simulink subsystem "PvtSubSys_VSM_ISL"  (R2020b)
settings: Solver=VariableStepAuto  StartTime=0.0  StopTime=10.0  RelTol=1e-3
values from neighbouring files (symbols this model uses):
  P_VSM_ISL_AutoSpPpercentage = 0.1    [ISL.sldd]
  P_VSM_ISL_SLW_Warning_Time = 10.0    [ISL.sldd]
  P_VSM_ISL_SpdDOWNmaxDiff = 50.0    [ISL.sldd]
  P_VSM_ISL_SpdUPmaxDiff = 25.0    [ISL.sldd]
  P_VSM_ISL_SpdUPminDiff = 10.0    [ISL.sldd]
  P_VSM_ISL_TimeInformDis = 6.0    [ISL.sldd]
  P_VSM_ISL_TimeTakeOver = 30.0    [ISL.sldd]
undefined symbols (not defined in the file or in its folder): ACC_STATE, HWA_STATE, TJA_STATE
libraries: simulink x17
settings Model: Creator=GW00133806  LastModifiedBy=Cheng

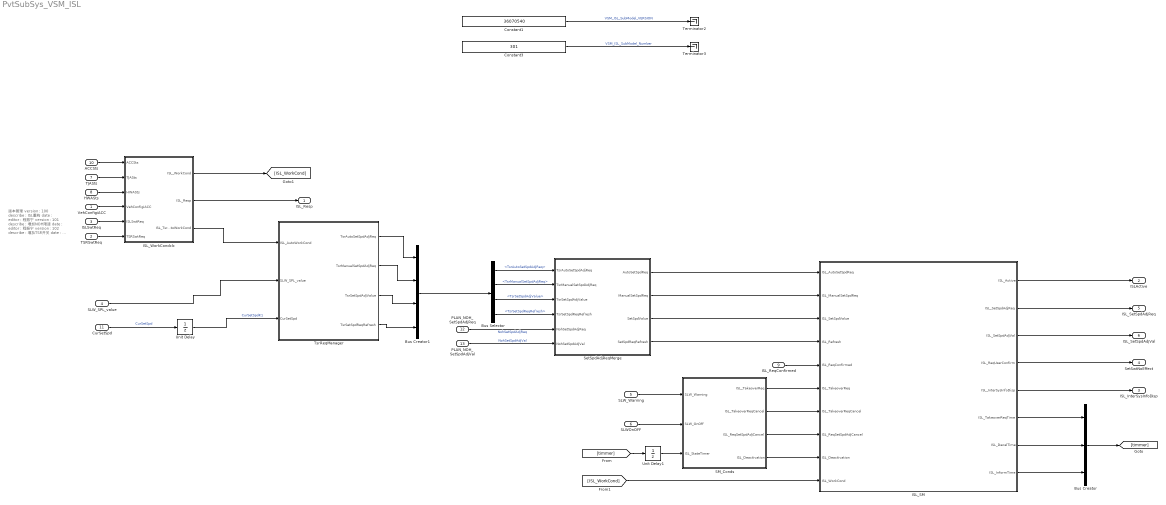
== system PvtSubSys_VSM_ISL ==
  note: 版本管理
      | version：100
      | describe：ISL重构
      | date：
      | editor：程振宁
      |
      | version：101
      | describe：增加NOH限速
      | date：
      | editor：程振宁
      |
      | version：102
      | describe：增加TSR开关
      | date：
      | editor：胡振国
  VehConfigiACC : Inport  OutDataTypeStr=uint8
  TSRSwtReq : Inport  Port=2
  ISLSwtReq : Inport  Port=3  OutDataTypeStr=boolean
  SLW_SPL_value : Inport  Port=4  OutDataTypeStr=uint8
  SLW_Warning : Inport  Port=5  OutDataTypeStr=boolean
  SLWOnOFF : Inport  Port=6  OutDataTypeStr=boolean
  TJASts : Inport  Port=7  OutDataTypeStr=Enum: TJA_STATE
  HWASts : Inport  Port=8  OutDataTypeStr=Enum: HWA_STATE
  ISL_ReqConfirmed : Inport  Port=9  OutDataTypeStr=boolean
  ACCSts : Inport  Port=10  OutDataTypeStr=Enum: ACC_STATE
  CurSetSpd : Inport  Port=11  OutDataTypeStr=single
  PLAN_NOH_SetSpdAdjReq : Inport  Port=12  OutDataTypeStr=boolean
  PLAN_NOH_SetSpdAdjVal : Inport  Port=13  OutDataTypeStr=uint8
  Bus Creator : BusCreator  Inputs=3
  Bus Creator1 : BusCreator  Inputs=4
  Bus Selector : BusSelector  OutputSignals=TsrAutoSetSpdAdjReq,TsrManualSetSpdAdjReq,TsrSetSpdAdjValue,TsrSetSpdReqRefresh
  Constant1 : Constant  Value=36070540  OutDataTypeStr=uint32
  Constant3 : Constant  Value=301  OutDataTypeStr=uint16
  ISL_SM : Stateflow chart  TreatAsAtomicUnit=on
  ISL_WorkCondclc : Subsystem
  SM_Conds : Subsystem
  SetSpdAdjReqMerge : Subsystem
  Terminator2 : Terminator
  Terminator3 : Terminator
  TsrReqManager : Subsystem
  Unit Delay : UnitDelay  SampleTime=-1  HasFrameUpgradeWarning=on
  Unit Delay1 : UnitDelay  SampleTime=-1  HasFrameUpgradeWarning=on
  ISL_Resp : Outport  OutDataTypeStr=boolean
  ISLActive : Outport  Port=2  OutDataTypeStr=boolean
  ISL_InterSysInfoDisp : Outport  Port=3  OutDataTypeStr=uint8
  SetSwtNoEffect : Outport  Port=4  OutDataTypeStr=boolean
  ISL_SetSpdAdjReq : Outport  Port=5  OutDataTypeStr=boolean
  ISL_SetSpdAdjVal : Outport  Port=6  OutDataTypeStr=uint8
  wires:
  Constant3/1 -> Terminator3/1  "VSM_ISL_SubModel_Number"
  Constant1/1 -> Terminator2/1  "VSM_ISL_SubModel_VERSION"
  TSRSwtReq/1 -> ISL_WorkCondclc/6(TSRSwtReq)
  Bus Selector/4 -> SetSpdAdjReqMerge/4(TsrSetSpdReqRefresh)  "<TsrSetSpdReqRefresh>"
  Bus Selector/3 -> SetSpdAdjReqMerge/3(TsrSetSpdAdjValue)  "<TsrSetSpdAdjValue>"
  Bus Selector/2 -> SetSpdAdjReqMerge/2(TsrManualSetSpdAdjReq)  "<TsrManualSetSpdAdjReq>"
  Bus Selector/1 -> SetSpdAdjReqMerge/1(TsrAutoSetSpdAdjReq)  "<TsrAutoSetSpdAdjReq>"
  SetSpdAdjReqMerge/4(SetSpdReqRefresh) -> ISL_SM/4(ISL_Refresh)
  SetSpdAdjReqMerge/3(SetSpdValue) -> ISL_SM/3(ISL_SetSpdValue)
  SetSpdAdjReqMerge/2(ManualSetSpdReq) -> ISL_SM/2(ISL_ManualSetSpdReq)
  SetSpdAdjReqMerge/1(AutoSetSpdReq) -> ISL_SM/1(ISL_AutoSetSpdReq)
  [ISL_WorkCond] -> ISL_SM/10(ISL_WorkCond)
  Bus Creator1/1 -> Bus Selector/1
  TsrReqManager/4(TsrSetSpdReqRefresh) -> Bus Creator1/4
  TsrReqManager/3(TsrSetSpdAdjValue) -> Bus Creator1/3
  TsrReqManager/2(TsrManualSetSpdAdjReq) -> Bus Creator1/2
  TsrReqManager/1(TsrAutoSetSpdAdjReq) -> Bus Creator1/1
  SM_Conds/4(ISL_Deactivation) -> ISL_SM/9(ISL_Deactivation)
  SM_Conds/3(ISL_ReqSetSpdAdjCancel) -> ISL_SM/8(ISL_ReqSetSpdAdjCancel)
  SM_Conds/2(ISL_TakeoverReqCancel) -> ISL_SM/7(ISL_TakeoverReqCancel)
  SM_Conds/1(ISL_TakeoverReq) -> ISL_SM/6(ISL_TakeoverReq)
  ISL_ReqConfirmed/1 -> ISL_SM/5(ISL_ReqConfirmed)
  Unit Delay1/1 -> SM_Conds/3(ISL_StateTimer)
  Bus Creator/1 -> [timmer]
  PLAN_NOH_SetSpdAdjVal/1 -> SetSpdAdjReqMerge/6(NohSetSpdAdjVal)  "NohSetSpdAdjVal"
  PLAN_NOH_SetSpdAdjReq/1 -> SetSpdAdjReqMerge/5(NohSetSpdAdjReq)  "NohSetSpdAdjReq"
  CurSetSpd/1 -> Unit Delay/1  "CurSetSpd"
  ISL_WorkCondclc/2(ISL_Resp) -> ISL_Resp/1
  SLW_Warning/1 -> SM_Conds/1(SLW_Warning)
  ISL_SM/4(ISL_ReqUserConfirm) -> SetSwtNoEffect/1
  VehConfigiACC/1 -> ISL_WorkCondclc/4(VehConfigiACC)
  SLW_SPL_value/1 -> TsrReqManager/2(SLW_SPL_value)
  ACCSts/1 -> ISL_WorkCondclc/1(ACCSts)
  ISL_SM/6(ISL_TakeoverReqTime) -> Bus Creator/1
  Unit Delay/1 -> TsrReqManager/3(CurSetSpd)  "CurSetSpdK1"
  ISL_SM/7(ISL_DecelTime) -> Bus Creator/2
  ISL_SM/5(ISL_InterSysInfoDisp) -> ISL_InterSysInfoDisp/1
  ISL_WorkCondclc/3(ISL_TsrAutoWorkCond) -> TsrReqManager/1(ISL_AutoWorkCond)
  ISL_SM/1(ISL_Active) -> ISLActive/1
  ISL_SM/2(ISL_SetSpdAdjReq) -> ISL_SetSpdAdjReq/1
  SLWOnOFF/1 -> SM_Conds/2(SLW_OnOff)
  ISL_SM/3(ISL_SetSpdAdjVal) -> ISL_SetSpdAdjVal/1
  ISLSwtReq/1 -> ISL_WorkCondclc/5(ISLSwtReq)
  HWASts/1 -> ISL_WorkCondclc/3(HWASts)
  ISL_WorkCondclc/1(ISL_WorkCond) -> [ISL_WorkCond]
  TJASts/1 -> ISL_WorkCondclc/2(TJASts)
  ISL_SM/8(ISL_InformTime) -> Bus Creator/3
  [timmer] -> Unit Delay1/1

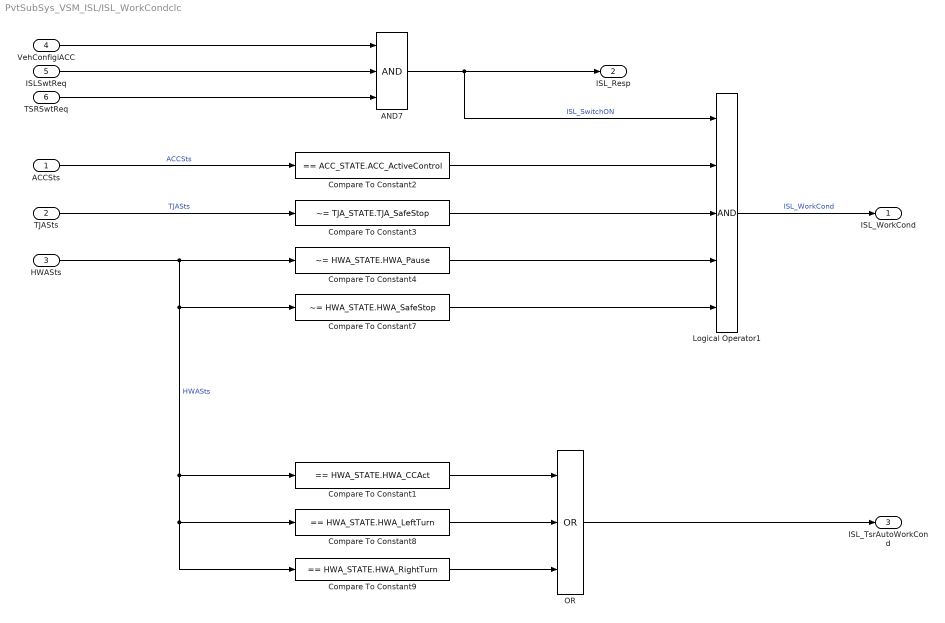
== system PvtSubSys_VSM_ISL/ISL_WorkCondclc ==
  ACCSts : Inport
  TJASts : Inport  Port=2
  HWASts : Inport  Port=3
  VehConfigiACC : Inport  Port=4
  ISLSwtReq : Inport  Port=5  OutDataTypeStr=boolean
  TSRSwtReq : Inport  Port=6
  AND7 : Logic  Inputs=3  AllPortsSameDT=off  OutDataTypeStr=boolean
  Compare To Constant1 : simulink/Logic and Bit Operations/Compare To Constant  relop===  const=HWA_STATE.HWA_CCAct  OutDataTypeStr=boolean
  Compare To Constant2 : simulink/Logic and Bit Operations/Compare To Constant  relop===  const=ACC_STATE.ACC_ActiveControl  OutDataTypeStr=boolean
  Compare To Constant3 : simulink/Logic and Bit Operations/Compare To Constant  relop=~=  const=TJA_STATE.TJA_SafeStop  OutDataTypeStr=boolean
  Compare To Constant4 : simulink/Logic and Bit Operations/Compare To Constant  relop=~=  const=HWA_STATE.HWA_Pause  OutDataTypeStr=boolean
  Compare To Constant7 : simulink/Logic and Bit Operations/Compare To Constant  relop=~=  const=HWA_STATE.HWA_SafeStop  OutDataTypeStr=boolean
  Compare To Constant8 : simulink/Logic and Bit Operations/Compare To Constant  relop===  const=HWA_STATE.HWA_LeftTurn  OutDataTypeStr=boolean
  Compare To Constant9 : simulink/Logic and Bit Operations/Compare To Constant  relop===  const=HWA_STATE.HWA_RightTurn  OutDataTypeStr=boolean
  Logical Operator1 : Logic  Inputs=5  AllPortsSameDT=off  OutDataTypeStr=boolean
  OR : Logic  Operator=OR  Inputs=3  AllPortsSameDT=off  OutDataTypeStr=boolean
  ISL_WorkCond : Outport
  ISL_Resp : Outport  Port=2
  ISL_TsrAutoWorkCond : Outport  Port=3
  wires:
  ACCSts/1 -> Compare To Constant2/1  "ACCSts"
  TJASts/1 -> Compare To Constant3/1  "TJASts"
  Compare To Constant2/1 -> Logical Operator1/2
  HWASts/1 -> Compare To Constant4/1, Compare To Constant9/1, Compare To Constant8/1, Compare To Constant1/1, Compare To Constant7/1  "HWASts"
  Logical Operator1/1 -> ISL_WorkCond/1  "ISL_WorkCond"
  Compare To Constant7/1 -> Logical Operator1/5
  Compare To Constant3/1 -> Logical Operator1/3
  Compare To Constant4/1 -> Logical Operator1/4
  TSRSwtReq/1 -> AND7/3
  ISLSwtReq/1 -> AND7/2
  AND7/1 -> Logical Operator1/1, ISL_Resp/1  "ISL_SwitchON"
  VehConfigiACC/1 -> AND7/1
  Compare To Constant1/1 -> OR/1
  Compare To Constant8/1 -> OR/2
  Compare To Constant9/1 -> OR/3
  OR/1 -> ISL_TsrAutoWorkCond/1

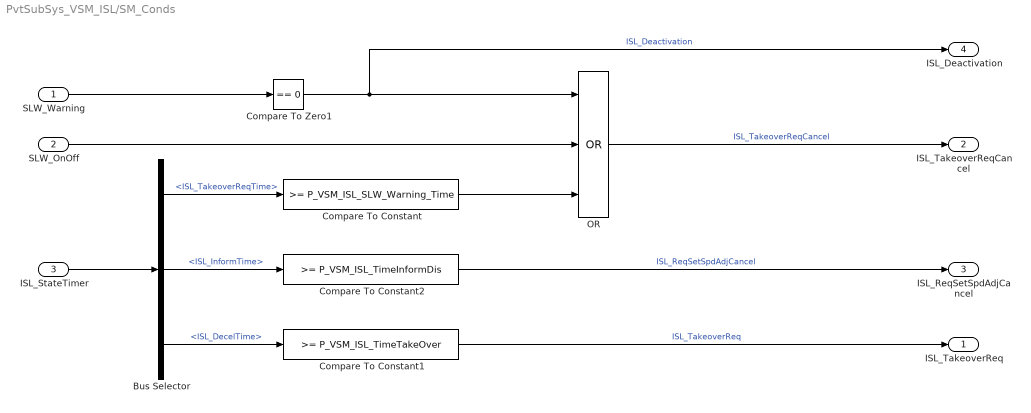
== system PvtSubSys_VSM_ISL/SM_Conds ==
  SLW_Warning : Inport
  SLW_OnOff : Inport  Port=2
  ISL_StateTimer : Inport  Port=3
  Bus Selector : BusSelector  OutputSignals=ISL_TakeoverReqTime,ISL_InformTime,ISL_DecelTime
  Compare To Constant : simulink/Logic and Bit Operations/Compare To Constant  relop=>=  const=P_VSM_ISL_SLW_Warning_Time  OutDataTypeStr=boolean
  Compare To Constant1 : simulink/Logic and Bit Operations/Compare To Constant  relop=>=  const=P_VSM_ISL_TimeTakeOver  OutDataTypeStr=boolean
  Compare To Constant2 : simulink/Logic and Bit Operations/Compare To Constant  relop=>=  const=P_VSM_ISL_TimeInformDis  OutDataTypeStr=boolean
  Compare To Zero1 : simulink/Logic and Bit Operations/Compare To Zero  relop===  OutDataTypeStr=boolean
  OR : Logic  Operator=OR  Inputs=3  AllPortsSameDT=off  OutDataTypeStr=boolean
  ISL_TakeoverReq : Outport
  ISL_TakeoverReqCancel : Outport  Port=2
  ISL_ReqSetSpdAdjCancel : Outport  Port=3
  ISL_Deactivation : Outport  Port=4
  wires:
  Compare To Constant1/1 -> ISL_TakeoverReq/1  "ISL_TakeoverReq"
  Bus Selector/1 -> Compare To Constant/1  "<ISL_TakeoverReqTime>"
  Compare To Constant/1 -> OR/3
  SLW_OnOff/1 -> OR/2
  SLW_Warning/1 -> Compare To Zero1/1
  OR/1 -> ISL_TakeoverReqCancel/1  "ISL_TakeoverReqCancel"
  Compare To Zero1/1 -> OR/1, ISL_Deactivation/1  "ISL_Deactivation"
  Bus Selector/2 -> Compare To Constant2/1  "<ISL_InformTime>"
  Compare To Constant2/1 -> ISL_ReqSetSpdAdjCancel/1  "ISL_ReqSetSpdAdjCancel"
  Bus Selector/3 -> Compare To Constant1/1  "<ISL_DecelTime>"
  ISL_StateTimer/1 -> Bus Selector/1

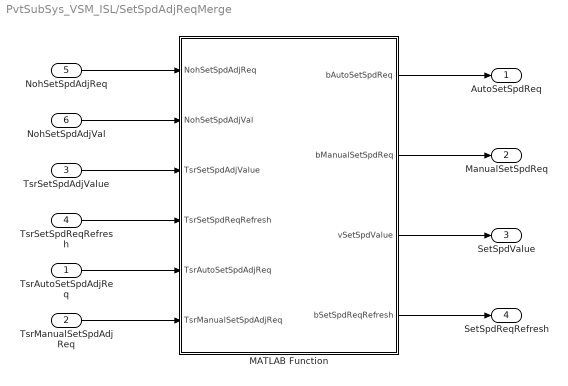
== system PvtSubSys_VSM_ISL/SetSpdAdjReqMerge ==
  TsrAutoSetSpdAdjReq : Inport
  TsrManualSetSpdAdjReq : Inport  Port=2
  TsrSetSpdAdjValue : Inport  Port=3
  TsrSetSpdReqRefresh : Inport  Port=4
  NohSetSpdAdjReq : Inport  Port=5
  NohSetSpdAdjVal : Inport  Port=6
  MATLAB Function : MATLAB Function  TreatAsAtomicUnit=on
  AutoSetSpdReq : Outport
  ManualSetSpdReq : Outport  Port=2
  SetSpdValue : Outport  Port=3
  SetSpdReqRefresh : Outport  Port=4
  wires:
  NohSetSpdAdjReq/1 -> MATLAB Function/1(NohSetSpdAdjReq)
  NohSetSpdAdjVal/1 -> MATLAB Function/2(NohSetSpdAdjVal)
  TsrSetSpdAdjValue/1 -> MATLAB Function/3(TsrSetSpdAdjValue)
  TsrSetSpdReqRefresh/1 -> MATLAB Function/4(TsrSetSpdReqRefresh)
  TsrAutoSetSpdAdjReq/1 -> MATLAB Function/5(TsrAutoSetSpdAdjReq)
  TsrManualSetSpdAdjReq/1 -> MATLAB Function/6(TsrManualSetSpdAdjReq)
  MATLAB Function/1(bAutoSetSpdReq) -> AutoSetSpdReq/1
  MATLAB Function/2(bManualSetSpdReq) -> ManualSetSpdReq/1
  MATLAB Function/3(vSetSpdValue) -> SetSpdValue/1
  MATLAB Function/4(bSetSpdReqRefresh) -> SetSpdReqRefresh/1

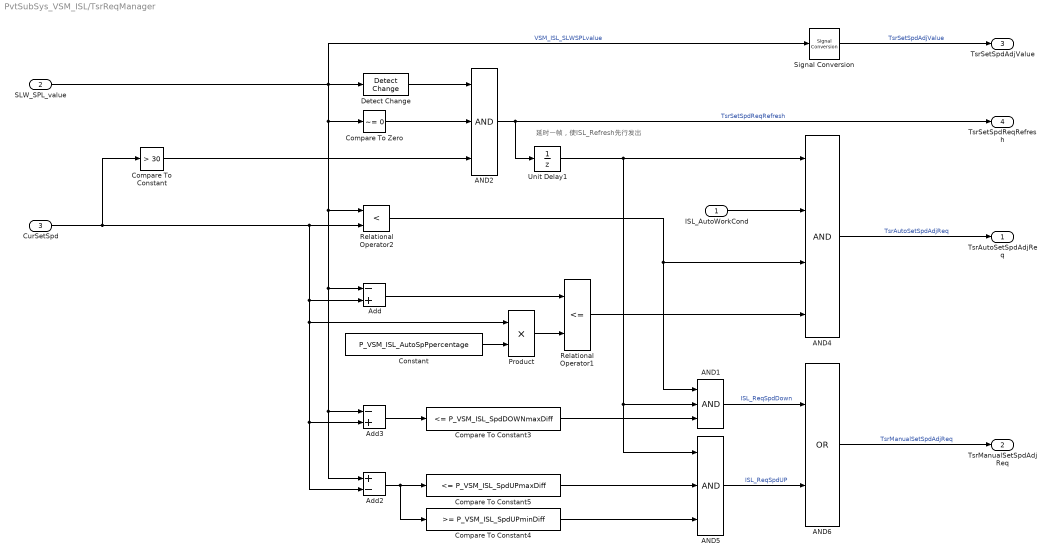
== system PvtSubSys_VSM_ISL/TsrReqManager ==
  note: 延时一帧，使ISL_Refresh先行发出
  ISL_AutoWorkCond : Inport
  SLW_SPL_value : Inport  Port=2
  CurSetSpd : Inport  Port=3
  AND1 : Logic  Inputs=3  AllPortsSameDT=off  OutDataTypeStr=boolean
  AND2 : Logic  Inputs=3  AllPortsSameDT=off  OutDataTypeStr=boolean
  AND4 : Logic  Inputs=4  AllPortsSameDT=off  OutDataTypeStr=boolean
  AND5 : Logic  Inputs=3  AllPortsSameDT=off  OutDataTypeStr=boolean
  AND6 : Logic  Operator=OR  AllPortsSameDT=off  OutDataTypeStr=boolean
  Add : Sum  Inputs=-+
  Add2 : Sum  Inputs=+-
  Add3 : Sum  Inputs=-+
  Compare To Constant : simulink/Logic and Bit Operations/Compare To Constant  relop=>  const=30  OutDataTypeStr=boolean
  Compare To Constant3 : simulink/Logic and Bit Operations/Compare To Constant  relop=<=  const=P_VSM_ISL_SpdDOWNmaxDiff  OutDataTypeStr=boolean
  Compare To Constant4 : simulink/Logic and Bit Operations/Compare To Constant  relop=>=  const=P_VSM_ISL_SpdUPminDiff  OutDataTypeStr=boolean
  Compare To Constant5 : simulink/Logic and Bit Operations/Compare To Constant  relop=<=  const=P_VSM_ISL_SpdUPmaxDiff  OutDataTypeStr=boolean
  Compare To Zero : simulink/Logic and Bit Operations/Compare To Zero  relop=~=  OutDataTypeStr=boolean
  Constant : Constant  Value=P_VSM_ISL_AutoSpPpercentage
  Detect Change : simulink/Logic and Bit Operations/Detect Change  vinit=0  OutDataTypeStr=boolean
  Product : Product
  Relational Operator1 : RelationalOperator  Operator=<=  OutDataTypeStr=boolean  RndMeth=Simplest
  Relational Operator2 : RelationalOperator  Operator=<  OutDataTypeStr=boolean  RndMeth=Simplest
  Signal Conversion : SignalConversion  OverrideOpt=off
  Unit Delay1 : UnitDelay  SampleTime=-1  HasFrameUpgradeWarning=on
  TsrAutoSetSpdAdjReq : Outport
  TsrManualSetSpdAdjReq : Outport  Port=2
  TsrSetSpdAdjValue : Outport  Port=3
  TsrSetSpdReqRefresh : Outport  Port=4
  wires:
  ISL_AutoWorkCond/1 -> AND4/2
  Relational Operator2/1 -> AND1/1, AND4/3
  Unit Delay1/1 -> AND5/1, AND1/2, AND4/1
  Constant/1 -> Product/2
  Product/1 -> Relational Operator1/2
  AND2/1 -> Unit Delay1/1, TsrSetSpdReqRefresh/1  "TsrSetSpdReqRefresh"
  AND6/1 -> TsrManualSetSpdAdjReq/1  "TsrManualSetSpdAdjReq"
  CurSetSpd/1 -> Compare To Constant/1, Add2/2, Add3/2, Product/1, Add/2, Relational Operator2/2
  AND1/1 -> AND6/1  "ISL_ReqSpdDown"
  Compare To Constant3/1 -> AND1/3
  Add3/1 -> Compare To Constant3/1
  AND5/1 -> AND6/2  "ISL_ReqSpdUP"
  Compare To Constant4/1 -> AND5/3
  Compare To Constant5/1 -> AND5/2
  Add2/1 -> Compare To Constant4/1, Compare To Constant5/1
  SLW_SPL_value/1 -> Signal Conversion/1, Add2/1, Add3/1, Add/1, Relational Operator2/1, Compare To Zero/1, Detect Change/1  "VSM_ISL_SLWSPLvalue"
  AND4/1 -> TsrAutoSetSpdAdjReq/1  "TsrAutoSetSpdAdjReq"
  Relational Operator1/1 -> AND4/4
  Add/1 -> Relational Operator1/1
  Detect Change/1 -> AND2/1
  Compare To Zero/1 -> AND2/2
  Signal Conversion/1 -> TsrSetSpdAdjValue/1  "TsrSetSpdAdjValue"
  Compare To Constant/1 -> AND2/3

== matlab function PvtSubSys_VSM_ISL/SetSpdAdjReqMerge/MATLAB Function ==
  data: NohSetSpdAdjReq input; bAutoSetSpdReq output; NohSetSpdAdjVal input; TsrSetSpdAdjValue input; TsrSetSpdReqRefresh input; TsrAutoSetSpdAdjReq input; TsrManualSetSpdAdjReq input; bManualSetSpdReq output; vSetSpdValue output; bSetSpdReqRefresh output
function [bAutoSetSpdReq,bManualSetSpdReq, vSetSpdValue, bSetSpdReqRefresh] ...
    = fcn(NohSetSpdAdjReq, NohSetSpdAdjVal, TsrSetSpdAdjValue, TsrSetSpdReqRefresh, TsrAutoSetSpdAdjReq, TsrManualSetSpdAdjReq)
if NohSetSpdAdjReq
    bAutoSetSpdReq=false;
    bManualSetSpdReq=true;
    vSetSpdValue=NohSetSpdAdjVal;
else
    if TsrManualSetSpdAdjReq
        bAutoSetSpdReq=false;
        bManualSetSpdReq=true;
        vSetSpdValue=TsrSetSpdAdjValue;
    elseif TsrAutoSetSpdAdjReq
        bAutoSetSpdReq=true;
        bManualSetSpdReq=false;
        vSetSpdValue=TsrSetSpdAdjValue;
    else
        bAutoSetSpdReq=false;
        bManualSetSpdReq=false;
        vSetSpdValue=0x0;
    end
end
bSetSpdReqRefresh = TsrSetSpdReqRefresh;
end

== stateflow chart PvtSubSys_VSM_ISL/ISL_SM ==
  state ISLoff
  state ISLon
    state ISL_Standby
      ISL_InterSysInfoDisp=0;
      ISL_Active=false;
      ISL_SetSpdAdjReq=false;
      ISL_SetSpdAdjVal=uint8(0);
    state ISL_Work
      state ISL_Inform
        en:
        ISL_InformTime=0;
        ISL_InterSysInfoDisp=1;%请求确认
        ISL_ReqUserConfirm=true;
        du:
        ISL_InformTime...
        =min(ISL_InformTime+0.02,200);
        ex:
        ISL_InterSysInfoDisp=0;
        ISL_ReqUserConfirm=false;
        ISL_InformTime=0;
      state ISL_SpeedAdj
        ISL_SetSpdAdjReq=true;
        ISL_SetSpdAdjVal=targetSpd;
        ex:
        ISL_SetSpdAdjReq=false;
        ISL_SetSpdAdjVal=uint8(0);
      state ISL_Active
        en:
        ISL_DecelTime=0;
        ISL_Active=true;%抑制超速报警
        du:
        ISL_DecelTime...
        =min(ISL_DecelTime+0.02,200);
        ex:
        ISL_DecelTime=0;
        ISL_Active=false;
      state ISL_TakeoverReq
        en:
        ISL_TakeoverReqTime=0;
        du:
        ISL_InterSysInfoDisp=2;%takeoverreq
        ISL_TakeoverReqTime...
        =min(ISL_TakeoverReqTime+0.02,200);
        ex:
        ISL_TakeoverReqTime=0;
      ISL_Inform -> ISL_SpeedAdj [order 1] : [ISL_ReqConfirmed]
      ISL_SpeedAdj -> ISL_Active
      ISL_Active -> ISL_TakeoverReq [order 1] : [ISL_TakeoverReq]
    (default) -> ISL_Standby
    ISL_Work -> ISL_Standby : [ISL_Refresh]
    ISL_Inform -> ISL_Standby [order 2] : [ISL_ReqSetSpdAdjCancel]
    ISL_Standby -> ISL_Inform [order 2] : [ISL_ManualSetSpdReq]
        | {targetSpd=ISL_SetSpdValue;}
    ISL_Standby -> ISL_SpeedAdj [order 1] : [ISL_AutoSetSpdReq]
        | {targetSpd=ISL_SetSpdValue;}
    ISL_Active -> ISL_Standby [order 2] : [ISL_Deactivation]
    ISL_TakeoverReq -> ISL_Standby : [ISL_TakeoverReqCancel]
  (default) -> ISLoff
  ISLoff -> ISLon : [ISL_WorkCond]
  ISLon -> ISLoff : [~ISL_WorkCond]
  data: ISL_AutoSetSpdReq input boolean size=1; ISL_ManualSetSpdReq input boolean size=1; ISL_SetSpdValue input uint8 size=1; ISL_Refresh input boolean size=1; ISL_ReqConfirmed input boolean size=1; ISL_TakeoverReq input boolean size=1; ISL_TakeoverReqCancel input boolean size=1; ISL_ReqSetSpdAdjCancel input boolean size=1; ISL_Active output boolean size=1; ISL_SetSpdAdjReq output boolean size=1; ISL_SetSpdAdjVal output uint8 size=1; ISL_ReqUserConfirm output boolean size=1; ISL_InterSysInfoDisp output uint8 size=1; ISL_TakeoverReqTime output single size=1; ISL_DecelTime output single size=1; ISL_InformTime output single size=1; ISL_Deactivation input; ISL_WorkCond input; targetSpd local
